simulink subsystem "Battery_Model"  (R2024a)
settings: Solver=VariableStepAuto  StartTime=0.0  StopTime=10.0  RelTol=1e-3
undefined symbols (not defined in the file): Battery, Np_Module
libraries: fl_lib x580, nesl_utility x386, batteryecm_lib x96, simulink x96
(part 3 of 6)

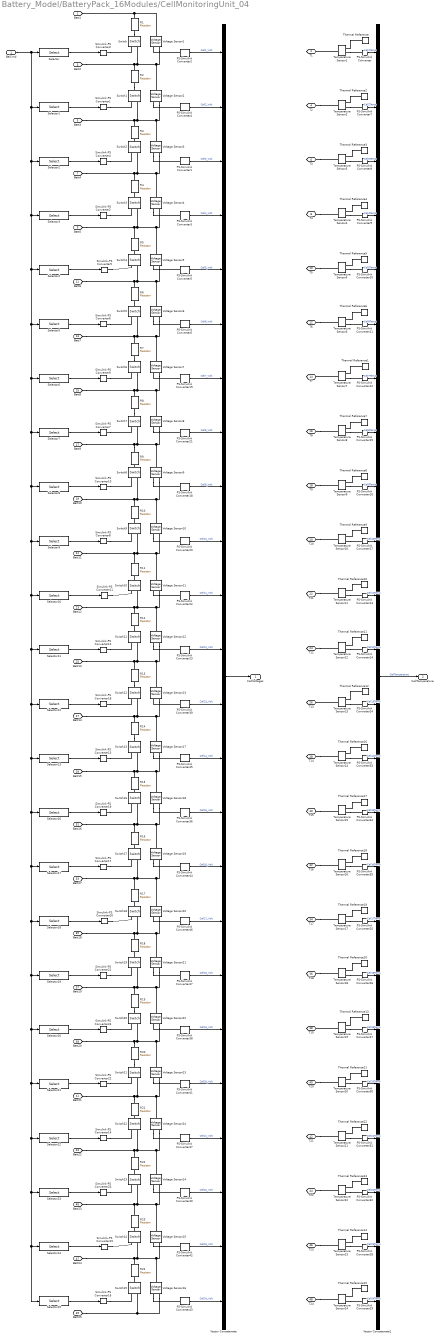
== system Battery_Model/BatteryPack_16Modules/CellMonitoringUnit_04 ==
  BalCmd : Inport
  PS-Simulink Converter{,7..17,24..35} (24 alike) : nesl_utility/PS-Simulink Converter  PhysicalDomain=network_engine_domain  SubClassName=ps_output  LeftPortType=input  RightPortType=output  PseudoPeriodic=off  Frequencies=[]  VectorFormat=1-D array  Unit=degC  AffineConversion=on
  PS-Simulink Converter{1..6,18..23,36..47} (24 alike) : nesl_utility/PS-Simulink Converter  PhysicalDomain=network_engine_domain  SubClassName=ps_output  LeftPortType=input  RightPortType=output  PseudoPeriodic=off  Frequencies=[]  VectorFormat=1-D array  Unit=V  AffineConversion=off
  R{1..24} (24 alike) : fl_lib/Electrical/Electrical Elements/Resistor  R=Battery.R_bleed Ohm  i_specify=off  i_priority=None  i=0 A  i_nominal_specify=off  i_nominal_value=1  i_nominal_unit=A  v_specify=off  v_priority=None  v=0 V  v_nominal_specify=off  v_nominal_value=1  v_nominal_unit=V
      R1 settings: LogSimulationData=on
      R13 settings: LogSimulationData=on
      R19 settings: LogSimulationData=on
      R7 settings: LogSimulationData=on
  Selector : Selector  IndexOptions=Index vector (dialog)  Indices=1  OutputSizes=1
  Selector1 : Selector  IndexOptions=Index vector (dialog)  Indices=2  OutputSizes=1
  Selector10 : Selector  IndexOptions=Index vector (dialog)  Indices=11  OutputSizes=1
  Selector11 : Selector  IndexOptions=Index vector (dialog)  Indices=12  OutputSizes=1
  Selector12 : Selector  IndexOptions=Index vector (dialog)  Indices=13  OutputSizes=1
  Selector13 : Selector  IndexOptions=Index vector (dialog)  Indices=14  OutputSizes=1
  Selector14 : Selector  IndexOptions=Index vector (dialog)  Indices=23  OutputSizes=1
  Selector15 : Selector  IndexOptions=Index vector (dialog)  Indices=24  OutputSizes=1
  Selector16 : Selector  IndexOptions=Index vector (dialog)  Indices=15  OutputSizes=1
  Selector17 : Selector  IndexOptions=Index vector (dialog)  Indices=16  OutputSizes=1
  Selector18 : Selector  IndexOptions=Index vector (dialog)  Indices=17  OutputSizes=1
  Selector19 : Selector  IndexOptions=Index vector (dialog)  Indices=18  OutputSizes=1
  Selector2 : Selector  IndexOptions=Index vector (dialog)  Indices=3  OutputSizes=1
  Selector20 : Selector  IndexOptions=Index vector (dialog)  Indices=19  OutputSizes=1
  Selector21 : Selector  IndexOptions=Index vector (dialog)  Indices=20  OutputSizes=1
  Selector22 : Selector  IndexOptions=Index vector (dialog)  Indices=21  OutputSizes=1
  Selector23 : Selector  IndexOptions=Index vector (dialog)  Indices=22  OutputSizes=1
  Selector3 : Selector  IndexOptions=Index vector (dialog)  Indices=4  OutputSizes=1
  Selector4 : Selector  IndexOptions=Index vector (dialog)  Indices=5  OutputSizes=1
  Selector5 : Selector  IndexOptions=Index vector (dialog)  Indices=6  OutputSizes=1
  Selector6 : Selector  IndexOptions=Index vector (dialog)  Indices=7  OutputSizes=1
  Selector7 : Selector  IndexOptions=Index vector (dialog)  Indices=8  OutputSizes=1
  Selector8 : Selector  IndexOptions=Index vector (dialog)  Indices=9  OutputSizes=1
  Selector9 : Selector  IndexOptions=Index vector (dialog)  Indices=10  OutputSizes=1
  Simulink-PS Converter{1..24} (24 alike) : nesl_utility/Simulink-PS Converter  PhysicalDomain=network_engine_domain  SubClassName=ps_input  LeftPortType=input  RightPortType=output  PseudoPeriodic=off  Frequencies=[]  NoiseDistribution=none  NoiseParameters=[]  Unit=1  AffineConversion=off  FilteringAndDerivatives=zero  SimscapeFilterOrder=1  InputFilterTimeConstant=0.001  UdotUserProvided=1
  Switch{,1..23} (24 alike) : fl_lib/Electrical/Electrical Elements/Switch  R_closed=0.01 Ohm  G_open=1e-8 1/Ohm  Threshold=0  i_specify=off  i_priority=None  i=0 A  i_nominal_specify=off  i_nominal_value=1  i_nominal_unit=A  v_specify=off  v_priority=None  v=0 V  v_nominal_specify=off  v_nominal_value=1  v_nominal_unit=V
  Temperature Sensor{1..24} (24 alike) : fl_lib/Thermal/Thermal Sensors/Temperature Sensor  temperature_measure=foundation.enum.MeasurementReference.difference
  Thermal Reference{,1..23} (24 alike) : fl_lib/Thermal/Thermal Elements/Thermal Reference
  Vector Concatenate : Concatenate  NumInputs=24
  Vector Concatenate1 : Concatenate  NumInputs=24
  Voltage Sensor{1..24} (24 alike) : fl_lib/Electrical/Electrical Sensors/Voltage Sensor
  Batt1 : PMIOPort  Side=Left
  T1 : PMIOPort  Port=2  Side=Left
  Batt2 : PMIOPort  Port=3  Side=Left
  T2 : PMIOPort  Port=4  Side=Left
  Batt3 : PMIOPort  Port=5  Side=Left
  T3 : PMIOPort  Port=6  Side=Left
  Batt4 : PMIOPort  Port=7  Side=Left
  T4 : PMIOPort  Port=8  Side=Left
  Batt5 : PMIOPort  Port=9  Side=Left
  T5 : PMIOPort  Port=10  Side=Left
  Batt6 : PMIOPort  Port=11  Side=Left
  T6 : PMIOPort  Port=12  Side=Left
  Batt7 : PMIOPort  Port=13  Side=Left
  T7 : PMIOPort  Port=14  Side=Left
  Batt8 : PMIOPort  Port=15  Side=Left
  T8 : PMIOPort  Port=16  Side=Left
  Batt9 : PMIOPort  Port=17  Side=Left
  T9 : PMIOPort  Port=18  Side=Left
  Batt10 : PMIOPort  Port=19  Side=Left
  T10 : PMIOPort  Port=20  Side=Left
  Batt11 : PMIOPort  Port=21  Side=Left
  T11 : PMIOPort  Port=22  Side=Left
  Batt12 : PMIOPort  Port=23  Side=Left
  T12 : PMIOPort  Port=24  Side=Left
  Batt13 : PMIOPort  Port=25  Side=Left
  T13 : PMIOPort  Port=26  Side=Left
  Batt14 : PMIOPort  Port=27  Side=Left
  T14 : PMIOPort  Port=28  Side=Left
  Batt15 : PMIOPort  Port=29  Side=Left
  T15 : PMIOPort  Port=30  Side=Left
  Batt16 : PMIOPort  Port=31  Side=Left
  T16 : PMIOPort  Port=32  Side=Left
  Batt17 : PMIOPort  Port=33  Side=Left
  T17 : PMIOPort  Port=34  Side=Left
  Batt18 : PMIOPort  Port=35  Side=Left
  T18 : PMIOPort  Port=36  Side=Left
  Batt19 : PMIOPort  Port=37  Side=Left
  T19 : PMIOPort  Port=38  Side=Left
  Batt20 : PMIOPort  Port=39  Side=Left
  T20 : PMIOPort  Port=40  Side=Left
  Batt21 : PMIOPort  Port=41  Side=Left
  T21 : PMIOPort  Port=42  Side=Left
  Batt22 : PMIOPort  Port=43  Side=Left
  T22 : PMIOPort  Port=44  Side=Left
  Batt23 : PMIOPort  Port=45  Side=Left
  T23 : PMIOPort  Port=46  Side=Left
  Batt24 : PMIOPort  Port=47  Side=Left
  T24 : PMIOPort  Port=48  Side=Left
  Batt25 : PMIOPort  Port=49  Side=Left
  CellVoltages : Outport  VectorParamsAs1DForOutWhenUnconnected=off
  CellTemperature : Outport  Port=2  VectorParamsAs1DForOutWhenUnconnected=off
  wires:
  PS-Simulink Converter39/1 -> Vector Concatenate/13  "Cell13_Volt"
  Selector18/1 -> Simulink-PS Converter20/1
  PS-Simulink Converter45/1 -> Vector Concatenate/14  "Cell14_Volt"
  Selector23/1 -> Simulink-PS Converter23/1
  PS-Simulink Converter47/1 -> Vector Concatenate/18  "Cell18_Volt"
  PS-Simulink Converter40/1 -> Vector Concatenate/22  "Cell22_Volt"
  PS-Simulink Converter46/1 -> Vector Concatenate/17  "Cell17_Volt"
  Selector16/1 -> Simulink-PS Converter19/1
  PS-Simulink Converter42/1 -> Vector Concatenate/23  "Cell23_Volt"
  Selector21/1 -> Simulink-PS Converter22/1
  Selector14/1 -> Simulink-PS Converter15/1
  Selector22/1 -> Simulink-PS Converter14/1
  Selector20/1 -> Simulink-PS Converter24/1
  Selector15/1 -> Simulink-PS Converter16/1
  PS-Simulink Converter43/1 -> Vector Concatenate/24  "Cell24_Volt"
  PS-Simulink Converter41/1 -> Vector Concatenate/20  "Cell20_Volt"
  PS-Simulink Converter38/1 -> Vector Concatenate/19  "Cell19_Volt"
  PS-Simulink Converter37/1 -> Vector Concatenate/21  "Cell21_Volt"
  BalCmd/1 -> Selector3/1, Selector5/1, Selector9/1, Selector11/1, Selector12/1, Selector17/1, Selector19/1, Selector23/1, Selector15/1, Selector14/1, Selector22/1, Selector21/1, Selector20/1, Selector18/1, Selector16/1, Selector13/1, Selector10/1, Selector8/1, Selector7/1, Selector6/1, Selector4/1, Selector2/1, Selector1/1, Selector/1
  Selector13/1 -> Simulink-PS Converter13/1
  PS-Simulink Converter36/1 -> Vector Concatenate/15  "Cell15_Volt"
  Selector12/1 -> Simulink-PS Converter18/1
  Selector19/1 -> Simulink-PS Converter21/1
  Selector17/1 -> Simulink-PS Converter17/1
  PS-Simulink Converter44/1 -> Vector Concatenate/16  "Cell16_Volt"
  PS-Simulink Converter32/1 -> Vector Concatenate1/22  "Cell22Temp"
  PS-Simulink Converter35/1 -> Vector Concatenate1/16  "Cell16Temp"
  PS-Simulink Converter34/1 -> Vector Concatenate1/15  "Cell15Temp"
  PS-Simulink Converter26/1 -> Vector Concatenate1/18  "Cell18Temp"
  PS-Simulink Converter27/1 -> Vector Concatenate1/19  "Cell19Temp"
  PS-Simulink Converter29/1 -> Vector Concatenate1/24  "Cell24Temp"
  PS-Simulink Converter28/1 -> Vector Concatenate1/23  "Cell23Temp"
  PS-Simulink Converter31/1 -> Vector Concatenate1/21  "Cell21Temp"
  PS-Simulink Converter30/1 -> Vector Concatenate1/20  "Cell20Temp"
  PS-Simulink Converter25/1 -> Vector Concatenate1/17  "Cell17Temp"
  PS-Simulink Converter33/1 -> Vector Concatenate1/14  "Cell14Temp"
  PS-Simulink Converter24/1 -> Vector Concatenate1/13  "Cell13Temp"
  Selector10/1 -> Simulink-PS Converter11/1
  PS-Simulink Converter21/1 -> Vector Concatenate/8  "Cell8_Volt"
  PS-Simulink Converter19/1 -> Vector Concatenate/7  "Cell7_Volt"
  PS-Simulink Converter23/1 -> Vector Concatenate/12  "Cell12_Volt"
  PS-Simulink Converter22/1 -> Vector Concatenate/11  "Cell11_Volt"
  Selector7/1 -> Simulink-PS Converter7/1
  Selector8/1 -> Simulink-PS Converter10/1
  PS-Simulink Converter18/1 -> Vector Concatenate/9  "Cell9_Volt"
  Selector6/1 -> Simulink-PS Converter9/1
  Selector11/1 -> Simulink-PS Converter12/1
  Selector9/1 -> Simulink-PS Converter8/1
  PS-Simulink Converter20/1 -> Vector Concatenate/10  "Cell10_Volt"
  PS-Simulink Converter14/1 -> Vector Concatenate1/12  "Cell12Temp"
  PS-Simulink Converter16/1 -> Vector Concatenate1/9  "Cell9Temp"
  PS-Simulink Converter17/1 -> Vector Concatenate1/10  "Cell10Temp"
  PS-Simulink Converter13/1 -> Vector Concatenate1/11  "Cell11Temp"
  PS-Simulink Converter15/1 -> Vector Concatenate1/8  "Cell8Temp"
  PS-Simulink Converter12/1 -> Vector Concatenate1/7  "Cell7Temp"
  Vector Concatenate/1 -> CellVoltages/1
  Selector2/1 -> Simulink-PS Converter4/1
  Selector1/1 -> Simulink-PS Converter1/1
  Selector/1 -> Simulink-PS Converter3/1
  Selector3/1 -> Simulink-PS Converter2/1
  Selector4/1 -> Simulink-PS Converter5/1
  Selector5/1 -> Simulink-PS Converter6/1
  PS-Simulink Converter2/1 -> Vector Concatenate/1  "Cell1_Volt"
  PS-Simulink Converter4/1 -> Vector Concatenate/2  "Cell2_Volt"
  PS-Simulink Converter1/1 -> Vector Concatenate/3  "Cell3_Volt"
  PS-Simulink Converter3/1 -> Vector Concatenate/4  "Cell4_Volt"
  PS-Simulink Converter5/1 -> Vector Concatenate/5  "Cell5_Volt"
  PS-Simulink Converter6/1 -> Vector Concatenate/6  "Cell6_Volt"
  Vector Concatenate1/1 -> CellTemperature/1  "CellTemperature"
  PS-Simulink Converter/1 -> Vector Concatenate1/1  "Cell1Temp"
  PS-Simulink Converter9/1 -> Vector Concatenate1/4  "Cell4Temp"
  PS-Simulink Converter7/1 -> Vector Concatenate1/2  "Cell2Temp"
  PS-Simulink Converter8/1 -> Vector Concatenate1/3  "Cell3Temp"
  PS-Simulink Converter10/1 -> Vector Concatenate1/5  "Cell5Temp"
  PS-Simulink Converter11/1 -> Vector Concatenate1/6  "Cell6Temp"
  connections:
  Voltage Sensor24/RConn1 -- PS-Simulink Converter37/LConn1
  Simulink-PS Converter17/RConn1 -- Switch17/RConn1
  R20/RConn1 -- Switch21/LConn1
  R23/RConn1 -- Switch14/LConn1
  Simulink-PS Converter14/RConn1 -- Switch22/RConn1
  Simulink-PS Converter16/RConn1 -- Switch15/RConn1
  Simulink-PS Converter21/RConn1 -- Switch19/RConn1
  Voltage Sensor15/RConn1 -- PS-Simulink Converter42/LConn1
  R17/RConn1 -- Switch18/LConn1
  Simulink-PS Converter22/RConn1 -- Switch21/RConn1
  Simulink-PS Converter20/RConn1 -- Switch18/RConn1
  Switch19/LConn1 -- R18/RConn1
  Switch23/LConn1 -- R22/RConn1
  R19/RConn1 -- Switch20/LConn1
  Voltage Sensor16/RConn1 -- PS-Simulink Converter43/LConn1
  Voltage Sensor20/RConn1 -- PS-Simulink Converter46/LConn1
  Voltage Sensor14/RConn1 -- PS-Simulink Converter40/LConn1
  R15/RConn1 -- Switch16/LConn1
  R21/RConn1 -- Switch22/LConn1
  Switch17/LConn1 -- R16/RConn1
  Simulink-PS Converter13/RConn1 -- Switch13/RConn1
  Simulink-PS Converter18/RConn1 -- Switch12/RConn1
  Simulink-PS Converter24/RConn1 -- Switch20/RConn1
  PS-Simulink Converter38/LConn1 -- Voltage Sensor22/RConn1
  R13/RConn1 -- Switch12/LConn1
  Switch15/LConn1 -- R24/RConn1
  Voltage Sensor17/RConn1 -- PS-Simulink Converter45/LConn1
  Voltage Sensor18/RConn1 -- PS-Simulink Converter36/LConn1
  Voltage Sensor23/RConn1 -- PS-Simulink Converter41/LConn1
  Simulink-PS Converter23/RConn1 -- Switch23/RConn1
  Voltage Sensor19/RConn1 -- PS-Simulink Converter44/LConn1
  PS-Simulink Converter39/LConn1 -- Voltage Sensor13/RConn1
  R14/RConn1 -- Switch13/LConn1
  Voltage Sensor21/RConn1 -- PS-Simulink Converter47/LConn1
  Simulink-PS Converter15/RConn1 -- Switch14/RConn1
  Simulink-PS Converter19/RConn1 -- Switch16/RConn1
  Voltage Sensor16/RConn2 -- Switch15/RConn2 -- Batt25/RConn1
  R20/LConn1 -- Voltage Sensor23/LConn1 -- Voltage Sensor22/RConn2 -- Switch20/RConn2 -- Batt20/RConn1
  Voltage Sensor22/LConn1 -- Voltage Sensor21/RConn2 -- Switch19/RConn2 -- Batt19/RConn1 -- R19/LConn1
  Voltage Sensor17/RConn2 -- Batt15/RConn1 -- R15/LConn1 -- Switch13/RConn2 -- Voltage Sensor18/LConn1
  Batt17/RConn1 -- R17/LConn1 -- Voltage Sensor20/LConn1 -- Voltage Sensor19/RConn2 -- Switch17/RConn2
  Voltage Sensor17/LConn1 -- Voltage Sensor13/RConn2 -- Switch12/RConn2 -- Batt14/RConn1 -- R14/LConn1
  Switch23/RConn2 -- R23/LConn1 -- Batt23/RConn1 -- Voltage Sensor15/LConn1 -- Voltage Sensor14/RConn2
  R21/LConn1 -- Batt21/RConn1 -- Switch21/RConn2 -- Voltage Sensor23/RConn2 -- Voltage Sensor24/LConn1
  Voltage Sensor15/RConn2 -- Switch14/RConn2 -- Batt24/RConn1 -- R24/LConn1 -- Voltage Sensor16/LConn1
  Voltage Sensor18/RConn2 -- Batt16/RConn1 -- R16/LConn1 -- Switch16/RConn2 -- Voltage Sensor19/LConn1
  Voltage Sensor20/RConn2 -- Switch18/RConn2 -- Batt18/RConn1 -- R18/LConn1 -- Voltage Sensor21/LConn1
  Batt22/RConn1 -- R22/LConn1 -- Switch22/RConn2 -- Voltage Sensor14/LConn1 -- Voltage Sensor24/RConn2
  Temperature Sensor22/RConn2 -- PS-Simulink Converter32/LConn1
  Temperature Sensor20/RConn2 -- PS-Simulink Converter30/LConn1
  Thermal Reference21/LConn1 -- Temperature Sensor20/RConn1
  Temperature Sensor14/RConn2 -- PS-Simulink Converter33/LConn1
  Temperature Sensor19/RConn2 -- PS-Simulink Converter27/LConn1
  Temperature Sensor23/RConn2 -- PS-Simulink Converter28/LConn1
  Temperature Sensor19/LConn1 -- T19/RConn1
  T24/RConn1 -- Temperature Sensor24/LConn1
  T23/RConn1 -- Temperature Sensor23/LConn1
  T15/RConn1 -- Temperature Sensor15/LConn1
  T18/RConn1 -- Temperature Sensor18/LConn1
  T21/RConn1 -- Temperature Sensor21/LConn1
  Thermal Reference22/LConn1 -- Temperature Sensor21/RConn1
  Temperature Sensor24/RConn2 -- PS-Simulink Converter29/LConn1
  Temperature Sensor13/RConn2 -- PS-Simulink Converter24/LConn1
  Thermal Reference23/LConn1 -- Temperature Sensor22/RConn1
  T22/RConn1 -- Temperature Sensor22/LConn1
  T14/RConn1 -- Temperature Sensor14/LConn1
  Temperature Sensor18/RConn2 -- PS-Simulink Converter26/LConn1
  Thermal Reference12/LConn1 -- Temperature Sensor13/RConn1
  Thermal Reference15/LConn1 -- Temperature Sensor24/RConn1
  Thermal Reference14/LConn1 -- Temperature Sensor23/RConn1
  Thermal Reference13/LConn1 -- Temperature Sensor19/RConn1
  Temperature Sensor21/RConn2 -- PS-Simulink Converter31/LConn1
  Thermal Reference17/LConn1 -- Temperature Sensor15/RConn1
  Temperature Sensor15/RConn2 -- PS-Simulink Converter34/LConn1
  T20/RConn1 -- Temperature Sensor20/LConn1
  Thermal Reference16/LConn1 -- Temperature Sensor14/RConn1
  Temperature Sensor16/RConn2 -- PS-Simulink Converter35/LConn1
  Temperature Sensor17/RConn2 -- PS-Simulink Converter25/LConn1
  Temperature Sensor13/LConn1 -- T13/RConn1
  T17/RConn1 -- Temperature Sensor17/LConn1
  Thermal Reference19/LConn1 -- Temperature Sensor17/RConn1
  Thermal Reference18/LConn1 -- Temperature Sensor16/RConn1
  T16/RConn1 -- Temperature Sensor16/LConn1
  Thermal Reference20/LConn1 -- Temperature Sensor18/RConn1
  Simulink-PS Converter10/RConn1 -- Switch8/RConn1
  Switch11/LConn1 -- R12/RConn1
  Simulink-PS Converter12/RConn1 -- Switch11/RConn1
  R11/RConn1 -- Switch10/LConn1
  Simulink-PS Converter11/RConn1 -- Switch10/RConn1
  Simulink-PS Converter8/RConn1 -- Switch9/RConn1
  Voltage Sensor11/RConn1 -- PS-Simulink Converter22/LConn1
  R9/RConn1 -- Switch8/LConn1
  PS-Simulink Converter19/LConn1 -- Voltage Sensor7/RConn1
  Simulink-PS Converter9/RConn1 -- Switch6/RConn1
  Voltage Sensor9/RConn1 -- PS-Simulink Converter18/LConn1
  Voltage Sensor8/RConn1 -- PS-Simulink Converter21/LConn1
  R8/RConn1 -- Switch7/LConn1
  Voltage Sensor10/RConn1 -- PS-Simulink Converter20/LConn1
  Voltage Sensor12/RConn1 -- PS-Simulink Converter23/LConn1
  R7/RConn1 -- Switch6/LConn1
  Simulink-PS Converter7/RConn1 -- Switch7/RConn1
  Switch9/LConn1 -- R10/RConn1
  Voltage Sensor13/LConn1 -- Voltage Sensor12/RConn2 -- Switch11/RConn2 -- Batt13/RConn1 -- R13/LConn1
  R9/LConn1 -- Batt9/RConn1 -- Switch7/RConn2 -- Voltage Sensor8/RConn2 -- Voltage Sensor9/LConn1
  Batt11/RConn1 -- R11/LConn1 -- Voltage Sensor11/LConn1 -- Voltage Sensor10/RConn2 -- Switch9/RConn2
  Voltage Sensor11/RConn2 -- Switch10/RConn2 -- Batt12/RConn1 -- R12/LConn1 -- Voltage Sensor12/LConn1
  Voltage Sensor8/LConn1 -- Voltage Sensor7/RConn2 -- Switch6/RConn2 -- Batt8/RConn1 -- R8/LConn1
  Batt10/RConn1 -- R10/LConn1 -- Switch8/RConn2 -- Voltage Sensor10/LConn1 -- Voltage Sensor9/RConn2
  Thermal Reference8/LConn1 -- Temperature Sensor9/RConn1
  Temperature Sensor7/RConn2 -- PS-Simulink Converter12/LConn1
  T12/RConn1 -- Temperature Sensor12/LConn1
  Thermal Reference7/LConn1 -- Temperature Sensor8/RConn1
  T11/RConn1 -- Temperature Sensor11/LConn1
  T9/RConn1 -- Temperature Sensor9/LConn1
  Temperature Sensor7/LConn1 -- T7/RConn1
  T8/RConn1 -- Temperature Sensor8/LConn1
  Thermal Reference1/LConn1 -- Temperature Sensor7/RConn1
  Temperature Sensor12/RConn2 -- PS-Simulink Converter14/LConn1
  Thermal Reference10/LConn1 -- Temperature Sensor11/RConn1
  T10/RConn1 -- Temperature Sensor10/LConn1
  Thermal Reference11/LConn1 -- Temperature Sensor12/RConn1
  Temperature Sensor10/RConn2 -- PS-Simulink Converter17/LConn1
  Temperature Sensor9/RConn2 -- PS-Simulink Converter16/LConn1
  Thermal Reference9/LConn1 -- Temperature Sensor10/RConn1
  Temperature Sensor11/RConn2 -- PS-Simulink Converter13/LConn1
  Temperature Sensor8/RConn2 -- PS-Simulink Converter15/LConn1
  Voltage Sensor4/LConn1 -- Voltage Sensor3/RConn2 -- Batt4/RConn1 -- R4/LConn1 -- Switch2/RConn2
  Voltage Sensor3/RConn1 -- PS-Simulink Converter1/LConn1
  Simulink-PS Converter4/RConn1 -- Switch2/RConn1
  Simulink-PS Converter1/RConn1 -- Switch1/RConn1
  Simulink-PS Converter3/RConn1 -- Switch/RConn1
  R2/RConn1 -- Switch1/LConn1
  Voltage Sensor2/RConn1 -- PS-Simulink Converter4/LConn1
  PS-Simulink Converter2/LConn1 -- Voltage Sensor1/RConn1
  Batt1/RConn1 -- Voltage Sensor1/LConn1 -- R1/LConn1
  R3/RConn1 -- Switch2/LConn1
  R1/RConn1 -- Switch/LConn1
  Batt2/RConn1 -- Voltage Sensor2/LConn1 -- Voltage Sensor1/RConn2 -- Switch/RConn2 -- R2/LConn1
  Voltage Sensor3/LConn1 -- Batt3/RConn1 -- R3/LConn1 -- Switch1/RConn2 -- Voltage Sensor2/RConn2
  Voltage Sensor4/RConn2 -- Voltage Sensor5/LConn1 -- Switch3/RConn2 -- R5/LConn1 -- Batt5/RConn1
  Switch3/LConn1 -- R4/RConn1
  Simulink-PS Converter2/RConn1 -- Switch3/RConn1
  Switch4/RConn2 -- Batt6/RConn1 -- R6/LConn1 -- Voltage Sensor6/LConn1 -- Voltage Sensor5/RConn2
  Simulink-PS Converter5/RConn1 -- Switch4/RConn1
  R5/RConn1 -- Switch4/LConn1
  Voltage Sensor7/LConn1 -- Voltage Sensor6/RConn2 -- Switch5/RConn2 -- Batt7/RConn1 -- R7/LConn1
  Simulink-PS Converter6/RConn1 -- Switch5/RConn1
  Switch5/LConn1 -- R6/RConn1
  Voltage Sensor4/RConn1 -- PS-Simulink Converter3/LConn1
  Voltage Sensor5/RConn1 -- PS-Simulink Converter5/LConn1
  Voltage Sensor6/RConn1 -- PS-Simulink Converter6/LConn1
  Temperature Sensor3/RConn2 -- PS-Simulink Converter8/LConn1
  Temperature Sensor1/RConn2 -- PS-Simulink Converter/LConn1
  Temperature Sensor6/RConn2 -- PS-Simulink Converter11/LConn1
  Temperature Sensor4/RConn2 -- PS-Simulink Converter9/LConn1
  Thermal Reference3/LConn1 -- Temperature Sensor3/RConn1
  Temperature Sensor5/RConn2 -- PS-Simulink Converter10/LConn1
  Thermal Reference4/LConn1 -- Temperature Sensor4/RConn1
  Temperature Sensor2/RConn2 -- PS-Simulink Converter7/LConn1
  Thermal Reference6/LConn1 -- Temperature Sensor6/RConn1
  Thermal Reference2/LConn1 -- Temperature Sensor2/RConn1
  Thermal Reference5/LConn1 -- Temperature Sensor5/RConn1
  Temperature Sensor1/LConn1 -- T1/RConn1
  T2/RConn1 -- Temperature Sensor2/LConn1
  T3/RConn1 -- Temperature Sensor3/LConn1
  T4/RConn1 -- Temperature Sensor4/LConn1
  T5/RConn1 -- Temperature Sensor5/LConn1
  T6/RConn1 -- Temperature Sensor6/LConn1
  Thermal Reference/LConn1 -- Temperature Sensor1/RConn1

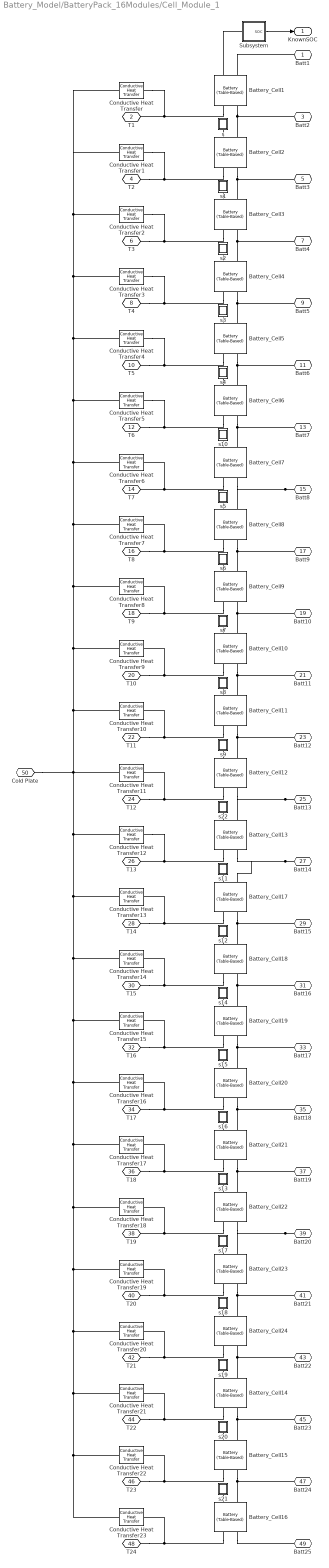
== system Battery_Model/BatteryPack_16Modules/Cell_Module_1 ==
  Battery_Cell{1..24} (24 alike) : batteryecm_lib/Battery (Table-Based)  Tag={'toolbox/physmod/elec/library/m/ee_lib_parts';'Sources/Battery__Table_Based_/Panasonic/NCR18650BD.xml'}  SOC_vec=Battery.SOC_LUT  T_dependence=simscape.enum.tablebattery.temperature_dependence.yes  prm_dir=simscape.enum.tablebattery.prm_dir.noCurrentDirectionality  T_vec=Battery.Temperature_LUT degC  V0_mat=Battery.Em_LUT V  V0_vec=[3.01162183959268 3.08575650269622 3.14177499163339 3.18631823552003 3.22334954767724 3.25390136234099 3.27878869705109 3.30070350874259 3.32118523630503 3.33873222862982 3.35681278765286 3.3727103181478 3.38793252475269 3.40246133852855 3.41323877471787 3.42274053961048 3.43230513033606 3.44127066639713 3.45046092538443 3.46050021597496 3.47059444208772 3.47754582201769 3.48403887676592 3.49083263175798 3.49762638675004 3.50414427848956 3.51006189737342 3.51650779121088 3.52300031605604 3.5294928409012 3.53574150484027 3.54126505716735 3.54599126111241 3.55084210438451 3.55569196094666 3.56052372392349 3.56532059653064 3.56979945432131 3.57444121267711 3.57904303346503 3.58364485425295 3.58840361874736 3.5931676308725 3.59914045642067 3.60536834334135 3.61166009904557 3.61797346412467 3.62428682920377 3.63060019428287 3.63762035332317 3.64493091713641 3.65193784155324 3.65894476597006 3.66595169038689 3.67346631195551 3.68205597286888 3.69093403907072 3.69981210527255 3.70876940774879 3.71776352136613 3.72686785650522 3.73538877817079 3.74389655120326 3.7524031927436 3.76046489817023 3.76888762106825 3.7779024493972 3.78684332393235 3.7957841984675 3.80453642296868 3.81235798589345 3.82032795054979 3.82829600796219 3.83626406537459 3.84436267545786 3.8525073311682 3.86057855536852 3.86864977956884 3.87672100376915 3.8849361052788 3.89310639828889 3.90173837211625 3.91095173577988 3.92144530461468 3.93240377767841 3.94373568413835 3.95558619350771 3.96743304428185 3.9792002957498 3.99089798499065 4.00334195302942 4.01527114968024 4.0272843604214 4.03909414300309 4.04916289177822 4.05870791988182 4.06775178122738 4.07651000374835 4.08674414955216 4.1040722856973] V  V_range=[0, inf] V  R0_mat=Battery.R0_LUT/Np_Module Ohm  R0_vec=[0.108383589577359 0.104276452250663 0.0975073630060557 0.0937501268832217 0.0893819468578965 0.085464471367626 0.08175755280038 0.0789657156023766 0.0763700410896049 0.0743500050394976 0.0728433546029721 0.0716898267238282 0.0709947524858037 0.0701675330798173 0.0687296636498531 0.0673712307537144 0.066215812656778 0.0650205672726791 0.0638581443118 0.0632667622677965 0.0628323749302964 0.0619127995096651 0.0610362875653991 0.0603620203223802 0.0596877530793609 0.0589554578065767 0.0582121279560432 0.0577538001128373 0.0573051863053595 0.0568565724978818 0.0563566623767877 0.055788965071129 0.0551527157042777 0.0546601636283963 0.0541676729953156 0.0536763090566326 0.0531776059040765 0.0526119236645948 0.0520712300263528 0.0515036752143958 0.0509361204024388 0.0503587926465561 0.0497811381187243 0.0494179007317461 0.0491061102549 0.0488178197046287 0.0485440631684004 0.0482703066321726 0.0479965500959447 0.0478381475470897 0.0477067926990284 0.0473712163371034 0.0470356399751788 0.0467000636132555 0.0464310667647791 0.0463210072143654 0.0462716139198203 0.0462222206252756 0.0462261199933538 0.0462489440940042 0.0463125045945074 0.0462585966454419 0.046201922872132 0.046144488080849 0.0458836890808221 0.0457208666912199 0.0456935258730669 0.0456707901856075 0.0456480544981481 0.0455856361429716 0.0453236882021848 0.0450859495122442 0.0448483295871047 0.0446107096619652 0.0444608967355156 0.0443618965142365 0.0442474499230245 0.0441330033318126 0.0440185567406002 0.0437935866730954 0.0434800673484186 0.0432636629093239 0.0431695542324042 0.0433145404237085 0.043616651255713 0.0439115402259742 0.0443155176840522 0.0447170344474341 0.0451426585495343 0.0455784262459233 0.0461653340876942 0.0463666936277911 0.0465478472510501 0.0466774333752156 0.0460938543815081 0.045231226285297 0.0442160431848739 0.0431407757562075 0.0415552249991693 0.0395514196760085] Ohm  R0_dis_mat=[0.03 0.015 0.002;0.04 0.017 0.008;0.039 0.012 0.006;0.027 0.013 0.021] % Parameter not set Ohm  R0_dis_vec=[0.015 0.017 0.012 0.013] % Parameter not set Ohm  R0_ch_mat=[0.03 0.015 0.002;0.04 0.017 0.008;0.039 0.012 0.006;0.027 0.013 0.021] % Parameter not set Ohm  R0_ch_vec=[0.015 0.017 0.012 0.013] % Parameter not set Ohm  AH=Battery.Capacity_LUT*Np_Module hr*A  prm_leak=simscape.enum.tablebattery.prm_leak.disabled  Rleak_vec=[8000 7000 6000] % Parameter not set Ohm  Rleak=7000 % Parameter not set Ohm  extrapolation_option=simscape.enum.extrapolation.nearest  SOC_port=simscape.enum.tablebattery.enable.yes  prm_dyn=simscape.enum.tablebattery.prm_dyn.rc1  R1_mat=Battery.R1_LUT/Np_Module Ohm  R1_vec=[0.076 0.022 0.007 0.043] % Parameter not set Ohm  tau1_mat=(Battery.R1_LUT/Np_Module).*(Battery.C1_LUT*Np_Module) s  tau1_vec=[148 110 27 22] % Parameter not set s  R2_mat=[0.014 0.382 0.407;0.028 0.006 0.007;0.014 0.007 0.006;0.333 0.956 0.912] % Parameter not set Ohm  R2_vec=[0.382 0.006 0.007 0.956] % Parameter not set Ohm  tau2_mat=[1 44 5644;11 24 506;2 14 330;3310 13419 30216] % Parameter not set s  tau2_vec=[44 24 14 13419] % Parameter not set s  R3_mat=[0.014 0.382 0.407;0.028 0.006 0.007;0.014 0.007 0.006;0.333 0.956 0.912] % Parameter not set Ohm  R3_vec=[0.382 0.006 0.007 0.956] % Parameter not set Ohm  tau3_mat=[1 44 5644;11 24 506;2 14 330;3310 13419 30216] % Parameter not set s  tau3_vec=[44 24 14 13419] % Parameter not set s  R4_mat=[0.014 0.382 0.407;0.028 0.006 0.007;0.014 0.007 0.006;0.333 0.956 0.912] % Parameter not set Ohm  R4_vec=[0.382 0.006 0.007 0.956] % Parameter not set Ohm  tau4_mat=[1 44 5644;11 24 506;2 14 330;3310 13419 30216] % Parameter not set s  tau4_vec=[44 24 14 13419] % Parameter not set s  R5_mat=[0.014 0.382 0.407;0.028 0.006 0.007;0.014 0.007 0.006;0.333 0.956 0.912] % Parameter not set Ohm  R5_vec=[0.382 0.006 0.007 0.956] % Parameter not set Ohm  tau5_mat=[1 44 5644;11 24 506;2 14 330;3310 13419 30216] % Parameter not set s  tau5_vec=[44 24 14 13419] % Parameter not set s  prm_fade=simscape.enum.tablebattery.prm_fade.tableN  N0=100 % Parameter not set  dV0=0 % Parameter not set  dR0=0 % Parameter not set  dAH=0 % Parameter not set  dRleak=0 % Parameter not set  dR1=0 % Parameter not set  dR2=0 % Parameter not set  dR3=0 % Parameter not set  dR4=0 % Parameter not set  dR5=0 % Parameter not set  N0vec=Battery.DischargeCycle_LUT  Tfadevec=[298.15 323.15] % Parameter not set K  dV0vec=Battery.deltaEm_LUT  dR0vec=[0;0;0;0;0;0;0;0;0;0;0;0;0;0;0;0;0;0;0;0;0;0;0;0;0;0;0;0;0;0;0;0;0;0;0;0;0;0;0;0;0;0;0;0;0;0;0;0;0;0;0;0;0;0;0;0;0;0;0;0;0;0;0;0;0;0;0;0;0;0;0;0;0;0;0;0;0;0;0;0] % Parameter not set  dAHvec=Battery.deltaCapacity_LUT  dRleakvec=[0 0 0] % Parameter not set  dR1vec=[0;0;0;0;0;0;0;0;0;0;0;0;0;0;0;0;0;0;0;0;0;0;0;0;0;0;0;0;0;0;0;0;0;0;0;0;0;0;0;0;0;0;0;0;0;0;0;0;0;0;0;0;0;0;0;0;0;0;0;0;0;0;0;0;0;0;0;0;0;0;0;0;0;0;0;0;0;0;0;0] % Parameter not set  dR2vec=[0 0 0] % Parameter not set  dR3vec=[0 0 0] % Parameter not set  dR4vec=[0 0 0] % Parameter not set  dR5vec=[0 0 0] % Parameter not set  dV0mat=[0 0;0 0;0 0] % Parameter not set  dR0mat=[0 0;0 0;0 0] % Parameter not set  dAHmat=[0 0;0 0;0 0] % Parameter not set  dRleakmat=[0 0;0 0;0 0] % Parameter not set  dR1mat=[0 0;0 0;0 0] % Parameter not set  dR2mat=[0 0;0 0;0 0] % Parameter not set  dR3mat=[0 0;0 0;0 0] % Parameter not set  dR4mat=[0 0;0 0;0 0] % Parameter not set  dR5mat=[0 0;0 0;0 0] % Parameter not set  prm_age_modeling=simscape.enum.tablebattery.prm_age_modeling.equation  storage_dt_age_vec=[0] d  storage_T_age_vec=[273] K  prm_age_OCV=simscape.enum.tablebattery.prm_age_OCV.OCV  OCV_age=0.9  SOC_age=0.6  prm_age_resistance=simscape.enum.tablebattery.prm_age.disabled  OCV_scaling_age_resistance=2.2134e6  OCV_offset_age_resistance=1.632e6  temp_exp_age_resistance=0.515833569 V  t_exp_age_resistance=0.75  T_age_vec_resistance=[273.15, 298.15, 323.15] K  dt_age_vec_resistance=[90, 180, 270, 360] d  dR0_age_vec=[0, 0, 0]  t_meas_dR0_age=100 d  dR0_age_mat=[0, 0, 0; 0, 0, 0; 0, 0, 0; 0, 0, 0]  prm_age_capacity=simscape.enum.tablebattery.prm_age.disabled  OCV_scaling_age_capacity=1.5097e07  OCV_offset_age_capacity=8.3625e06  temp_exp_age_capacity=0.6011 V  t_exp_age_capacity=0.75  T_age_vec_capacity=[273.15, 298.15, 323.15] K  dt_age_vec_capacity=[90, 180, 270, 360] d  dAH_age_vec=[0, 0, 0]  t_meas_dAH_age=100 d  dAH_age_mat=[0, 0, 0; 0, 0, 0; 0, 0, 0; 0, 0, 0]  thermal_port=simscape.enum.thermaleffects.model  temperature=BattTempInit degC  thermal_mass=Battery.ThermalMass*Np_Module J/K  i_specify=off  i_priority=None  i=0 A  i_nominal_specify=off  i_nominal_value=1  i_nominal_unit=A  v_specify=off  v_priority=None  v=0 V  v_nominal_specify=off  v_nominal_value=1  v_nominal_unit=V  stateOfCharge_specify=on  stateOfCharge_priority=High  stateOfCharge=BattSocInit  stateOfCharge_nominal_specify=off  stateOfCharge_nominal_value=1  stateOfCharge_nominal_unit=1  num_cycles_specify=off  num_cycles_priority=High  num_cycles=0  num_cycles_nominal_specify=off  num_cycles_nominal_value=1  num_cycles_nominal_unit=1  cell_temperature_specify=on  cell_temperature_priority=High  cell_temperature=BattTempInit degC  cell_temperature_nominal_specify=off  cell_temperature_nominal_value=1  cell_temperature_nominal_unit=K
      settings: AttributesFormatString=Panasonic:NCR18650BD
  Conductive Heat Transfer{,1..23} (24 alike) : fl_lib/Thermal/Thermal Elements/Conductive Heat Transfer  thermal_type=foundation.enum.ConstantVariableTabulated.Constant  wall_geometry=foundation.enum.ConductionWallGeometry.Planar  area=Battery.cell_area*Np_Module m^2  thickness=Battery.cond_thickness m  d_in=0.05 m  d_out=0.1 m  L=1 m  th_cond_min=10 W/(K*m)  th_cond=Battery.thermal_conductivity W/(m*K)  th_cond_TLU=[413, 401, 392, 383, 371, 357, 342] W/(K*m)  temp_TLU=[200, 273, 400, 600, 800, 1000, 1200] K  T_specify=off  T_priority=None  T=0 K  T_nominal_specify=off  T_nominal_value=1  T_nominal_unit=K  Q_specify=off  Q_priority=None  Q=0 W  Q_nominal_specify=off  Q_nominal_value=1  Q_nominal_unit=W
  Subsystem : Subsystem
  s : Subsystem
  s1 : Subsystem
  s10 : Subsystem
  s11 : Subsystem
  s12 : Subsystem
  s13 : Subsystem
  s14 : Subsystem
  s15 : Subsystem
  s16 : Subsystem
  s17 : Subsystem
  s18 : Subsystem
  s19 : Subsystem
  s2 : Subsystem
  s20 : Subsystem
  s21 : Subsystem
  s22 : Subsystem
  s3 : Subsystem
  s4 : Subsystem
  s5 : Subsystem
  s6 : Subsystem
  s7 : Subsystem
  s8 : Subsystem
  s9 : Subsystem
  Batt1 : PMIOPort  Side=Right
  T1 : PMIOPort  Port=2  Side=Right
  Batt2 : PMIOPort  Port=3  Side=Right
  T2 : PMIOPort  Port=4  Side=Right
  Batt3 : PMIOPort  Port=5  Side=Right
  T3 : PMIOPort  Port=6  Side=Right
  Batt4 : PMIOPort  Port=7  Side=Right
  T4 : PMIOPort  Port=8  Side=Right
  Batt5 : PMIOPort  Port=9  Side=Right
  T5 : PMIOPort  Port=10  Side=Right
  Batt6 : PMIOPort  Port=11  Side=Right
  T6 : PMIOPort  Port=12  Side=Right
  Batt7 : PMIOPort  Port=13  Side=Right
  T7 : PMIOPort  Port=14  Side=Right
  Batt8 : PMIOPort  Port=15  Side=Right
  T8 : PMIOPort  Port=16  Side=Right
  Batt9 : PMIOPort  Port=17  Side=Right
  T9 : PMIOPort  Port=18  Side=Right
  Batt10 : PMIOPort  Port=19  Side=Right
  T10 : PMIOPort  Port=20  Side=Right
  Batt11 : PMIOPort  Port=21  Side=Right
  T11 : PMIOPort  Port=22  Side=Right
  Batt12 : PMIOPort  Port=23  Side=Right
  T12 : PMIOPort  Port=24  Side=Right
  Batt13 : PMIOPort  Port=25  Side=Right
  T13 : PMIOPort  Port=26  Side=Right
  Batt14 : PMIOPort  Port=27  Side=Right
  T14 : PMIOPort  Port=28  Side=Right
  Batt15 : PMIOPort  Port=29  Side=Right
  T15 : PMIOPort  Port=30  Side=Right
  Batt16 : PMIOPort  Port=31  Side=Right
  T16 : PMIOPort  Port=32  Side=Right
  Batt17 : PMIOPort  Port=33  Side=Right
  T17 : PMIOPort  Port=34  Side=Right
  Batt18 : PMIOPort  Port=35  Side=Right
  T18 : PMIOPort  Port=36  Side=Right
  Batt19 : PMIOPort  Port=37  Side=Right
  T19 : PMIOPort  Port=38  Side=Right
  Batt20 : PMIOPort  Port=39  Side=Right
  T20 : PMIOPort  Port=40  Side=Right
  Batt21 : PMIOPort  Port=41  Side=Right
  T21 : PMIOPort  Port=42  Side=Right
  Batt22 : PMIOPort  Port=43  Side=Right
  T22 : PMIOPort  Port=44  Side=Right
  Batt23 : PMIOPort  Port=45  Side=Right
  T23 : PMIOPort  Port=46  Side=Right
  Batt24 : PMIOPort  Port=47  Side=Right
  T24 : PMIOPort  Port=48  Side=Right
  Batt25 : PMIOPort  Port=49  Side=Right
  Cold Plate : PMIOPort  Port=50  Side=Left
  KnownSOC : Outport
  wires:
  Subsystem/1(soc) -> KnownSOC/1
  connections:
  Battery_Cell13/LConn2 -- s22/LConn1
  Battery_Cell24/LConn2 -- s18/LConn1
  Battery_Cell16/RConn1 -- Batt25/RConn1
  Battery_Cell18/LConn2 -- s12/LConn1
  Battery_Cell22/LConn2 -- s13/LConn1
  Battery_Cell17/LConn2 -- s11/LConn1
  Battery_Cell15/LConn2 -- s20/LConn1
  Battery_Cell21/LConn2 -- s16/LConn1
  Battery_Cell23/LConn2 -- s17/LConn1
  Battery_Cell16/LConn2 -- s21/LConn1
  Battery_Cell19/LConn2 -- s14/LConn1
  Battery_Cell20/LConn2 -- s15/LConn1
  Battery_Cell14/LConn2 -- s19/LConn1
  Battery_Cell17/RConn1 -- Batt15/RConn1 -- Battery_Cell18/LConn1
  Battery_Cell15/RConn2 -- Conductive Heat Transfer22/LConn1 -- T23/RConn1
  Battery_Cell22/RConn2 -- Conductive Heat Transfer18/LConn1 -- T19/RConn1
  Battery_Cell21/RConn1 -- Batt19/RConn1 -- Battery_Cell22/LConn1
  Battery_Cell14/LConn1 -- Batt22/RConn1 -- Battery_Cell24/RConn1
  Battery_Cell20/RConn2 -- Conductive Heat Transfer16/LConn1 -- T17/RConn1
  Battery_Cell13/RConn2 -- Conductive Heat Transfer12/LConn1 -- T13/RConn1
  Battery_Cell18/RConn2 -- Conductive Heat Transfer14/LConn1 -- T15/RConn1
  Battery_Cell16/RConn2 -- Conductive Heat Transfer23/LConn1 -- T24/RConn1
  Battery_Cell14/RConn2 -- Conductive Heat Transfer21/LConn1 -- T22/RConn1
  Battery_Cell20/RConn1 -- Batt18/RConn1 -- Battery_Cell21/LConn1
  Battery_Cell14/RConn1 -- Batt23/RConn1 -- Battery_Cell15/LConn1
  Battery_Cell19/RConn1 -- Batt17/RConn1 -- Battery_Cell20/LConn1
  Battery_Cell23/RConn2 -- Conductive Heat Transfer19/LConn1 -- T20/RConn1
  Battery_Cell24/RConn2 -- Conductive Heat Transfer20/LConn1 -- T21/RConn1
  Battery_Cell17/RConn2 -- Conductive Heat Transfer13/LConn1 -- T14/RConn1
  Battery_Cell15/RConn1 -- Batt24/RConn1 -- Battery_Cell16/LConn1
  Battery_Cell19/LConn1 -- Batt16/RConn1 -- Battery_Cell18/RConn1
  Battery_Cell19/RConn2 -- Conductive Heat Transfer15/LConn1 -- T16/RConn1
  Battery_Cell23/RConn1 -- Batt21/RConn1 -- Battery_Cell24/LConn1
  Battery_Cell21/RConn2 -- Conductive Heat Transfer17/LConn1 -- T18/RConn1
  Batt14/RConn1 -- Battery_Cell17/LConn1 -- Battery_Cell13/RConn1
  Batt20/RConn1 -- Battery_Cell23/LConn1 -- Battery_Cell22/RConn1
  Battery_Cell7/LConn2 -- s10/LConn1
  Battery_Cell9/LConn2 -- s6/LConn1
  Battery_Cell8/LConn2 -- s5/LConn1
  Battery_Cell12/LConn2 -- s9/LConn1
  Battery_Cell10/LConn2 -- s7/LConn1
  Batt13/RConn1 -- Battery_Cell13/LConn1 -- Battery_Cell12/RConn1
  Battery_Cell11/LConn2 -- s8/LConn1
  Battery_Cell9/RConn2 -- Conductive Heat Transfer8/LConn1 -- T9/RConn1
  Battery_Cell8/RConn2 -- Conductive Heat Transfer7/LConn1 -- T8/RConn1
  Battery_Cell11/RConn2 -- Conductive Heat Transfer10/LConn1 -- T11/RConn1
  Battery_Cell10/LConn1 -- Batt10/RConn1 -- Battery_Cell9/RConn1
  Battery_Cell10/RConn1 -- Batt11/RConn1 -- Battery_Cell11/LConn1
  Battery_Cell10/RConn2 -- Conductive Heat Transfer9/LConn1 -- T10/RConn1
  Battery_Cell8/RConn1 -- Batt9/RConn1 -- Battery_Cell9/LConn1
  Battery_Cell11/RConn1 -- Batt12/RConn1 -- Battery_Cell12/LConn1
  Battery_Cell12/RConn2 -- Conductive Heat Transfer11/LConn1 -- T12/RConn1
  Batt8/RConn1 -- Battery_Cell7/RConn1 -- Battery_Cell8/LConn1
  Battery_Cell7/RConn2 -- Conductive Heat Transfer6/LConn1 -- T7/RConn1
  Batt5/RConn1 -- Battery_Cell5/LConn1 -- Battery_Cell4/RConn1
  Batt6/RConn1 -- Battery_Cell6/LConn1 -- Battery_Cell5/RConn1
  Batt4/RConn1 -- Battery_Cell3/RConn1 -- Battery_Cell4/LConn1
  Battery_Cell1/RConn2 -- Conductive Heat Transfer/LConn1 -- T1/RConn1
  Battery_Cell5/RConn2 -- Conductive Heat Transfer4/LConn1 -- T5/RConn1
  Battery_Cell1/RConn1 -- Battery_Cell2/LConn1 -- Batt2/RConn1
  Battery_Cell6/RConn2 -- Conductive Heat Transfer5/LConn1 -- T6/RConn1
  Conductive Heat Transfer22/RConn1 -- Conductive Heat Transfer23/RConn1 -- Conductive Heat Transfer21/RConn1 -- Conductive Heat Transfer20/RConn1 -- Conductive Heat Transfer19/RConn1 -- Conductive Heat Transfer18/RConn1 -- Conductive Heat Transfer17/RConn1 -- Conductive Heat Transfer16/RConn1 -- Conductive Heat Transfer15/RConn1 -- Conductive Heat Transfer14/RConn1 -- Conductive Heat Transfer13/RConn1 -- Conductive Heat Transfer11/RConn1 -- Cold Plate/RConn1 -- Conductive Heat Transfer10/RConn1 -- Conductive Heat Transfer9/RConn1 -- Conductive Heat Transfer8/RConn1 -- Conductive Heat Transfer7/RConn1 -- Conductive Heat Transfer6/RConn1 -- Conductive Heat Transfer5/RConn1 -- Conductive Heat Transfer4/RConn1 -- Conductive Heat Transfer/RConn1 -- Conductive Heat Transfer1/RConn1 -- Conductive Heat Transfer2/RConn1 -- Conductive Heat Transfer3/RConn1 -- Conductive Heat Transfer12/RConn1
  Battery_Cell7/LConn1 -- Batt7/RConn1 -- Battery_Cell6/RConn1
  Batt1/RConn1 -- Battery_Cell1/LConn1
  Batt3/RConn1 -- Battery_Cell3/LConn1 -- Battery_Cell2/RConn1
  Battery_Cell1/LConn2 -- Subsystem/LConn1
  Battery_Cell2/LConn2 -- s/LConn1
  Battery_Cell3/LConn2 -- s1/LConn1
  Battery_Cell4/LConn2 -- s2/LConn1
  Battery_Cell5/LConn2 -- s3/LConn1
  Battery_Cell6/LConn2 -- s4/LConn1
  Battery_Cell3/RConn2 -- Conductive Heat Transfer2/LConn1 -- T3/RConn1
  Battery_Cell2/RConn2 -- Conductive Heat Transfer1/LConn1 -- T2/RConn1
  Battery_Cell4/RConn2 -- Conductive Heat Transfer3/LConn1 -- T4/RConn1
